simulink model "mypid"  (R2025a)
settings: Solver=FixedStepDiscrete  StartTime=0.0  StopTime=400  FixedStep=0.5  RelTol=1e-3
undefined symbols (not defined in the file): DiscIntNeverNeededParam
libraries: simulink x1
settings Model: Creator=bsb  LastModifiedBy=bsb

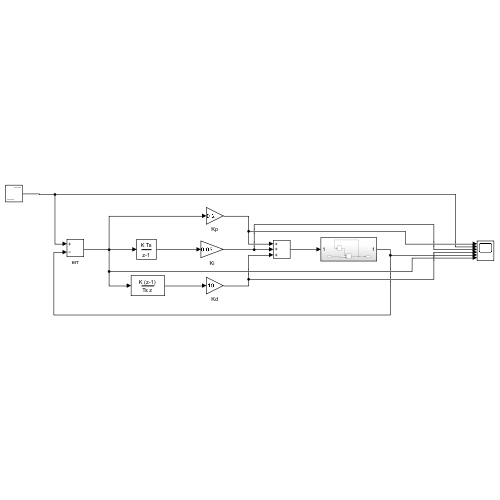
[thumbnail: Simulink's stored preview of the top-level diagram]
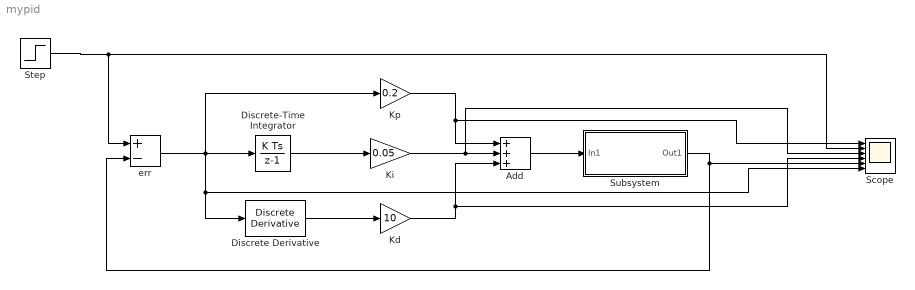
== system mypid ==
  Add : Sum  Inputs=+++
  Discrete Derivative : simulink/Discrete/Discrete Derivative  gainval=1.0  ICPrevScaledInput=0.0  OutMin=[]  OutMax=[]  OutDataType=fixdt(1, 16)  OutScaling=2^-10  DoSatur=off
  Discrete-Time Integrator : DiscreteIntegrator  SampleTime=-1  ICPrevOutput=DiscIntNeverNeededParam  ICPrevScaledInput=DiscIntNeverNeededParam
  Kd : Gain  Gain=10
  Ki : Gain  Gain=0.05
  Kp : Gain  Gain=0.2
  Scope : Scope  NumInputPorts=6
      settings: ActiveDisplayYMinimum=2.8797496269520528  ActiveDisplayYMaximum=7.8848437445871813
  Step : Step  After=5
  Subsystem : Subsystem
  err : Sum  Inputs=+-
  wires:
  Step/1 -> err/1, Scope/2
  Kp/1 -> Add/1, Scope/1
  Kd/1 -> Add/3, Scope/4
  Discrete-Time Integrator/1 -> Ki/1
  Add/1 -> Subsystem/1(In1)
  err/1 -> Discrete-Time Integrator/1, Discrete Derivative/1, Scope/6, Kp/1
  Ki/1 -> Scope/3, Add/2
  Discrete Derivative/1 -> Kd/1
  Subsystem/1(Out1) -> err/2, Scope/5

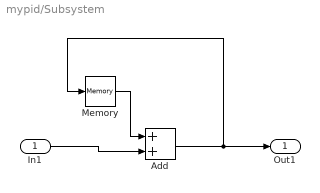
== system mypid/Subsystem ==
  In1 : Inport
  Add : Sum
  Memory : Memory  InheritSampleTime=on  LinearizeAsDelay=on
  Out1 : Outport
  wires:
  Memory/1 -> Add/1
  Add/1 -> Out1/1, Memory/1
  In1/1 -> Add/2
